simulink library "mcp2515lib"  (R2018b)
settings: Solver=VariableStepAuto  StartTime=0.0  StopTime=10.0  RelTol=1e-3  EnableMultiTasking=on
libraries: $bdroot x33, simulink x26, arduinolib x9, raspberrypilib x9
(part 1 of 2)
settings Model: Creator=ayasuda  LastModifiedBy=Tatsuya Ishikawa
settings DataIOCC: LimitDataPoints=on
settings OptimizationCC: LifeSpan=inf
settings DebuggingCC: UnderspecifiedInitializationDetection=Classic  MergeDetectMultiDrivingBlocksExec=none  AllowSymbolicDim=off  SFUnexpectedBacktrackingDiag=warning  SFNoUnconditionalDefaultTransitionDiag=warning  SFExecutionAtInitializationDiag=none
settings ModelReferenceCC: PropagateSignalLabelsOutOfModel=off
settings SFSimCC: SimUseLocalCustomCode=off
settings RTWCC: RTWUseLocalCustomCode=off
settings CodeAppCC: StateflowObjectComments=on
settings GRTTargetCC: TargetLangStandard=C89/C90 (ANSI)
settings ConfigComp: CovMetricSettings=dw  CovHtmlReporting=on  CovSaveCumulativeToWorkspaceVar=on  CovSaveSingleToWorkspaceVar=on  CovExternalEMLEnable=off

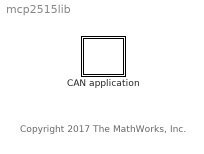
== system mcp2515lib ==
  note: Copyright 2017 The MathWorks, Inc.
  CAN application : Subsystem

== system mcp2515lib/CAN application ==
  note: Copyright 2017 The MathWorks, Inc.
  CANbegin : Subsystem  TreatAsAtomicUnit=on  mask{TargetHardware=Arduino, Oscillator=16, CANSpeed=1000, CSpin=10}
      mask prompts: TargetHardware "Target Hardware"; Oscillator "Oscillator frequency(MHz)"; CANSpeed "CAN speed(kHz)"; CSpin "Chip Select Pin"
      mask init:
      | % Get this mask's handle
      | maskObj = Simulink.Mask.get(gcb);
      | 
      | % Get the selected value from mask parameter's option
      | str_TargetHard = char(maskObj.Parameters(1).TypeOptions(TargetHardware));
      | str_Osc = char(maskObj.Parameters(2).TypeOptions(Oscillator));
      | str_CANSpeed = char(maskObj.Parameters(3).TypeOptions(CANSpeed));
      | 
      | % Set Icon
      | str1 = sprintf('%s(Model)',str_TargetHard);
      | str2 = sprintf('Oscillator: %s(MHz)',str_Osc);
      | str3 = sprintf('CAN Bus Speed: %s(kHz)',str_CANSpeed);
      | str4 = sprintf('Chip Select pin: %d',CSpin);
      | 
      | % Set the values of Variant Subsystem
      | switch str_TargetHard
      |     case 'Arduino'
      |         str = [str1,'\n',str2,'\n',str3,'\n',str4];
      |         evalin('base',sprintf('CSpin = %d;',CSpin));        
      |         evalin('base','Hardware = 1;');
      |     case 'Raspberry Pi'
      |         str = [str1,'\n',str2,'\n',str3];
      |         evalin('base',sprintf('clear CSpin',CSpin));           
      |         evalin('base','Hardware = 2;');     
      | end  
      | 
      | % Get the CAN Configuration register's value from mask parameter's option
      | if str_Osc == '8' %[MHz]
      |     switch str_CANSpeed
      |         case '1000'
      |             BPR = 0; PHSEG1 = 0; PRSEG = 0; PHSEG2 = 0;
      |         case '500'
      |             BPR = 0; PHSEG1 = 2; PRSEG = 0; PHSEG2 = 2;
      |         case '250'
      |             BPR = 0; PHSEG1 = 6; PRSEG = 0; PHSEG2 = 6;
      |         case '125'
      |             BPR = 1; PHSEG1 = 6; PRSEG = 1; PHSEG2 = 5;
      |         case '100'
      |             BPR = 1; PHSEG1 = 7; PRSEG = 2; PHSEG2 = 7;
      |         case '83.3'
      |             BPR = 1; PHSEG1 = 7; PRSEG = 6; PHSEG2 = 7;
      |         case '62.5'
      |             BPR = 3; PHSEG1 = 6; PRSEG = 0; PHSEG2 = 6;
      |         case '50'
      |             BPR = 3; PHSEG1 = 7; PRSEG = 2; PHSEG2 = 7;
      |         case '33.3'
      |             BPR = 4; PHSEG1 = 7; PRSEG = 6; PHSEG2 = 7;
      |     end            
      | elseif str_Osc == '16' %[MHz]
      |     switch str_CANSpeed  
      |         case '1000'
      |             BPR = 0; PHSEG1 = 2; PRSEG = 0; PHSEG2 = 2;
      |         case '500'
      |             BPR = 0; PHSEG1 = 6; PRSEG = 0; PHSEG2 = 6;
      |         case '250'
      |             BPR = 1; PHSEG1 = 6; PRSEG = 1; PHSEG2 = 5;        
      |         case '125'
      |             BPR = 3; PHSEG1 = 6; PRSEG = 0; PHSEG2 = 6;
      |         case '100'
      |             BPR = 3; PHSEG1 = 7; PRSEG = 2; PHSEG2 = 7;
      |         case '83.3'
      |             BPR = 3; PHSEG1 = 7; PRSEG = 6; PHSEG2 = 7;
      |         case '62.5'
      |             BPR = 7; PHSEG1 = 6; PRSEG = 0; PHSEG2 = 6;
      |         case '50'
      |             BPR = 7; PHSEG1 = 7; PRSEG = 2; PHSEG2 = 7;
      |         case '33.3'
      |             BPR = 9; PHSEG1 = 7; PRSEG = 6; PHSEG2 = 7;        
      |     end   
      | end
      | % Set the CAN Configuration register's value
      | address2A = BPR;          % bit7-6 :SJW, bit5-0: BPR
      | address29 = 192 ...       % bit7: BTLMODE = 1, bit6:SAM = 1
      |             + 8*PHSEG1 ...% bit5-3: PHSEG1
      |             +PRSEG;       % bit2-0: PRSEG
      | address28 = 128 ...       % bit7: SOF = 1, bit6:WAKFIL = 0
      |             + PHSEG2;     % bit5-3: 0, bit2-0: PHSEG2
      settings: OpenFcn=open_system(gcbh,'force')  RTWSystemCode=Nonreusable function
      settings: CopyFcn=|
      | set_param(gcbh,'LinkStatus','none');
      | set_param(gcbh,'OpenFcn','');
      | set_param(gcbh,'CopyFcn','')
      mask TypeOptions TargetHardware: Arduino | Raspberry Pi
      mask Callback TargetHardware:
      | if(strcmp(get_param(gcb,'TargetHardware'),'Arduino'))
      |     set_param(gcb,'MaskVisibilities',{'on','on','on','on'})
      | else
      |     set_param(gcb,'MaskVisibilities',{'on','on','on','off'})
      | end
      mask TypeOptions Oscillator: 8 | 16
      mask TypeOptions CANSpeed: 1000 | 500 | 250 | 125 | 100 | 83.3 | 62.5 | 50 | 33.3
      mask DialogControl DescGroupVar Prompt: Description
      mask DialogControl DescTextVar Prompt: This block must be executed only once when beginning CAN communication because MCP2515’s register needs to be configured. And the frequency of oscillator for MCP2515 is also needed because it effects to the setting parameters of MCP2515's register.
      mask Display: disp(str)
  CANbegin CE1 : Subsystem  TreatAsAtomicUnit=on  mask{TargetHardware=Arduino, Oscillator=8, CANSpeed=1000, CSpin=10}
      mask prompts: TargetHardware "Target Hardware"; Oscillator "Oscillator frequency(MHz)"; CANSpeed "CAN speed(kHz)"; CSpin "Chip Select Pin"
      mask init: same as mcp2515lib/CAN application/CANbegin
      settings: OpenFcn=open_system(gcbh,'force')  RTWSystemCode=Nonreusable function
      settings: CopyFcn=|
      | set_param(gcbh,'LinkStatus','none');
      | set_param(gcbh,'OpenFcn','');
      | set_param(gcbh,'CopyFcn','')
      mask TypeOptions TargetHardware: Arduino | Raspberry Pi
      mask Callback TargetHardware:
      | if(strcmp(get_param(gcb,'TargetHardware'),'Arduino'))
      |     set_param(gcb,'MaskVisibilities',{'on','on','on','on'})
      | else
      |     set_param(gcb,'MaskVisibilities',{'on','on','on','off'})
      | end
      mask TypeOptions Oscillator: 8 | 16
      mask TypeOptions CANSpeed: 1000 | 500 | 250 | 125 | 100 | 83.3 | 62.5 | 50 | 33.3
      mask DialogControl DescGroupVar Prompt: Description
      mask DialogControl DescTextVar Prompt: This block must be executed only once when beginning CAN communication because MCP2515’s register needs to be configured. And the frequency of oscillator for MCP2515 is also needed because it effects to the setting parameters of MCP2515's register.
      mask Display: disp(str)
  CANreceive : Subsystem  TreatAsAtomicUnit=on
      settings: OpenFcn=open_system(gcbh,'force')
      settings: CopyFcn=|
      | set_param(gcbh,'LinkStatus','none');
      | set_param(gcbh,'OpenFcn','');
      | set_param(gcbh,'CopyFcn','')
      mask DialogControl DescGroupVar Prompt: Description
      mask DialogControl DescTextVar Prompt: CANreceive outputs CAN data by converting MCP2515 RX buffer register’s values. In/Out ports are no use because they are used for controlling the execution order. CAN_Received outputs 1(CAN received) or -1( No message).
  CANreceive CE1 : Subsystem  TreatAsAtomicUnit=on
      settings: OpenFcn=open_system(gcbh,'force')
      settings: CopyFcn=|
      | set_param(gcbh,'LinkStatus','none');
      | set_param(gcbh,'OpenFcn','');
      | set_param(gcbh,'CopyFcn','')
      mask DialogControl DescGroupVar Prompt: Description
      mask DialogControl DescTextVar Prompt: CANreceive outputs CAN data by converting MCP2515 RX buffer register’s values. In/Out ports are no use because they are used for controlling the execution order. CAN_Received outputs 1(CAN received) or -1( No message).
  CANtransmit : Subsystem  TreatAsAtomicUnit=on
      settings: OpenFcn=open_system(gcbh,'force')
      settings: CopyFcn=|
      | set_param(gcbh,'LinkStatus','none');
      | set_param(gcbh,'OpenFcn','');
      | set_param(gcbh,'CopyFcn','')
      mask DialogControl DescGroupVar Prompt: Description
      mask DialogControl DescTextVar Prompt: CANtransmit inputs CAN data by converting MCP2515 TX buffer register’s values. In/Out ports are no use because they are used for controlling the execution order. CAN_Transmitted outputs 1(Success) or 2(Fail).
  CANtransmit CE1 : Subsystem  TreatAsAtomicUnit=on
      settings: OpenFcn=open_system(gcbh,'force')
      settings: CopyFcn=|
      | set_param(gcbh,'LinkStatus','none');
      | set_param(gcbh,'OpenFcn','');
      | set_param(gcbh,'CopyFcn','')
      mask DialogControl DescGroupVar Prompt: Description
      mask DialogControl DescTextVar Prompt: CANtransmit inputs CAN data by converting MCP2515 TX buffer register’s values. In/Out ports are no use because they are used for controlling the execution order. CAN_Transmitted outputs 1(Success) or 2(Fail).
  mcp2515 driver : Subsystem
  mcp2515 driver CE1 : Subsystem

== system mcp2515lib/CAN application/CANbegin ==
  Constant : Constant  Value=0  OutDataTypeStr=boolean  SampleTime=-1
  Temporary buffer : DataStoreMemory  DataStoreName=temp_1byte  ReadBeforeWriteMsg=warning  WriteAfterWriteMsg=warning  WriteAfterReadMsg=warning  ShowAdditionalParam=off  OutDataTypeStr=uint8
  Unit Delay : UnitDelay  InitialCondition=1  SampleTime=-1
  setup : Subsystem  TreatAsAtomicUnit=on
      settings: RTWSystemCode=Nonreusable function  RTWFileNameOpts=Use subsystem name
  wires:
  Constant/1 -> Unit Delay/1
  Unit Delay/1 -> setup/Enable

== system mcp2515lib/CAN application/CANbegin CE1 ==
  Constant : Constant  Value=0  OutDataTypeStr=boolean  SampleTime=-1
  Temporary buffer : DataStoreMemory  DataStoreName=temp_1byte  ReadBeforeWriteMsg=warning  WriteAfterWriteMsg=warning  WriteAfterReadMsg=warning  ShowAdditionalParam=off  OutDataTypeStr=uint8
  Unit Delay : UnitDelay  InitialCondition=1  SampleTime=-1
  setup : Subsystem  TreatAsAtomicUnit=on
      settings: RTWSystemCode=Nonreusable function  RTWFileNameOpts=Use subsystem name
  wires:
  Constant/1 -> Unit Delay/1
  Unit Delay/1 -> setup/Enable

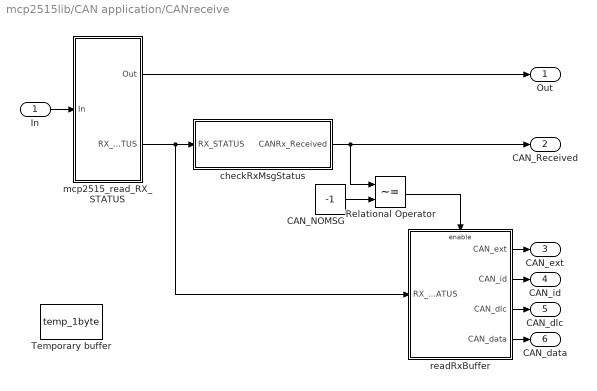
== system mcp2515lib/CAN application/CANreceive ==
  In : Inport
  CAN_NOMSG : Constant  Value=-1  OutDataTypeStr=int8
  Relational Operator : RelationalOperator  Operator=~=  OutDataTypeStr=boolean  RndMeth=Nearest
  Temporary buffer : DataStoreMemory  DataStoreName=temp_1byte  ReadBeforeWriteMsg=warning  WriteAfterWriteMsg=warning  WriteAfterReadMsg=warning  ShowAdditionalParam=off  OutDataTypeStr=uint8
  checkRxMsgStatus : Subsystem  TreatAsAtomicUnit=on
  mcp2515_read_RX_STATUS : Subsystem  TreatAsAtomicUnit=on
  readRxBuffer : Subsystem  TreatAsAtomicUnit=on
  Out : Outport
  CAN_Received : Outport  Port=2
  CAN_ext : Outport  Port=3
  CAN_id : Outport  Port=4
  CAN_dlc : Outport  Port=5
  CAN_data : Outport  Port=6
  wires:
  Relational Operator/1 -> readRxBuffer/Enable
  CAN_NOMSG/1 -> Relational Operator/2
  readRxBuffer/4(CAN_data) -> CAN_data/1
  readRxBuffer/3(CAN_dlc) -> CAN_dlc/1
  readRxBuffer/2(CAN_id) -> CAN_id/1
  readRxBuffer/1(CAN_ext) -> CAN_ext/1
  mcp2515_read_RX_STATUS/2(RX_STATUS) -> checkRxMsgStatus/1(RX_STATUS), readRxBuffer/1(RX_STATUS)
  checkRxMsgStatus/1(CANRx_Received) -> Relational Operator/1, CAN_Received/1
  mcp2515_read_RX_STATUS/1(Out) -> Out/1
  In/1 -> mcp2515_read_RX_STATUS/1(In)

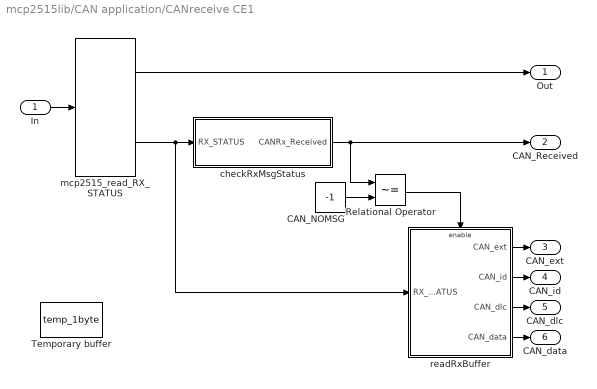
== system mcp2515lib/CAN application/CANreceive CE1 ==
  In : Inport
  CAN_NOMSG : Constant  Value=-1  OutDataTypeStr=int8
  Relational Operator : RelationalOperator  Operator=~=  OutDataTypeStr=boolean  RndMeth=Nearest
  Temporary buffer : DataStoreMemory  DataStoreName=temp_1byte  ReadBeforeWriteMsg=warning  WriteAfterWriteMsg=warning  WriteAfterReadMsg=warning  ShowAdditionalParam=off  OutDataTypeStr=uint8
  checkRxMsgStatus : Subsystem  TreatAsAtomicUnit=on
  mcp2515_read_RX_STATUS : $bdroot/CAN application/mcp2515 driver CE1/mcp2515_read_RX_STATUS  SystemSampleTime=-1
  readRxBuffer : Subsystem  TreatAsAtomicUnit=on
  Out : Outport
  CAN_Received : Outport  Port=2
  CAN_ext : Outport  Port=3
  CAN_id : Outport  Port=4
  CAN_dlc : Outport  Port=5
  CAN_data : Outport  Port=6
  wires:
  Relational Operator/1 -> readRxBuffer/Enable
  CAN_NOMSG/1 -> Relational Operator/2
  readRxBuffer/4(CAN_data) -> CAN_data/1
  readRxBuffer/3(CAN_dlc) -> CAN_dlc/1
  readRxBuffer/2(CAN_id) -> CAN_id/1
  readRxBuffer/1(CAN_ext) -> CAN_ext/1
  mcp2515_read_RX_STATUS/2 -> checkRxMsgStatus/1(RX_STATUS), readRxBuffer/1(RX_STATUS)
  checkRxMsgStatus/1(CANRx_Received) -> Relational Operator/1, CAN_Received/1
  mcp2515_read_RX_STATUS/1 -> Out/1
  In/1 -> mcp2515_read_RX_STATUS/1

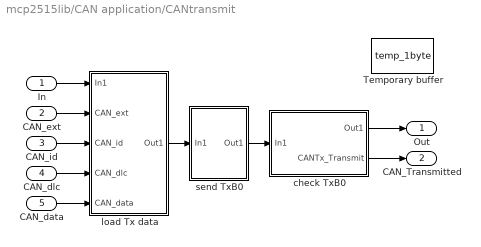
== system mcp2515lib/CAN application/CANtransmit ==
  In : Inport
  CAN_ext : Inport  Port=2
  CAN_id : Inport  Port=3
  CAN_dlc : Inport  Port=4
  CAN_data : Inport  Port=5
  Temporary buffer : DataStoreMemory  DataStoreName=temp_1byte  ReadBeforeWriteMsg=warning  WriteAfterWriteMsg=warning  WriteAfterReadMsg=warning  ShowAdditionalParam=off  OutDataTypeStr=uint8
  check TxB0 : Subsystem  TreatAsAtomicUnit=on
  load Tx data : Subsystem  TreatAsAtomicUnit=on
  send TxB0 : Subsystem  TreatAsAtomicUnit=on
  Out : Outport
  CAN_Transmitted : Outport  Port=2
  wires:
  CAN_data/1 -> load Tx data/5(CAN_data)
  CAN_dlc/1 -> load Tx data/4(CAN_dlc)
  CAN_id/1 -> load Tx data/3(CAN_id)
  CAN_ext/1 -> load Tx data/2(CAN_ext)
  check TxB0/2(CANTx_Transmit) -> CAN_Transmitted/1
  check TxB0/1(Out1) -> Out/1
  send TxB0/1(Out1) -> check TxB0/1(In1)
  load Tx data/1(Out1) -> send TxB0/1(In1)
  In/1 -> load Tx data/1(In1)

== system mcp2515lib/CAN application/CANtransmit CE1 ==
  In : Inport
  CAN_ext : Inport  Port=2
  CAN_id : Inport  Port=3
  CAN_dlc : Inport  Port=4
  CAN_data : Inport  Port=5
  Temporary buffer : DataStoreMemory  DataStoreName=temp_1byte  ReadBeforeWriteMsg=warning  WriteAfterWriteMsg=warning  WriteAfterReadMsg=warning  ShowAdditionalParam=off  OutDataTypeStr=uint8
  check TxB0 : Subsystem  TreatAsAtomicUnit=on
  load Tx data : Subsystem  TreatAsAtomicUnit=on
  send TxB0 : Subsystem  TreatAsAtomicUnit=on
  Out : Outport
  CAN_Transmitted : Outport  Port=2
  wires:
  CAN_data/1 -> load Tx data/5(CAN_data)
  CAN_dlc/1 -> load Tx data/4(CAN_dlc)
  CAN_id/1 -> load Tx data/3(CAN_id)
  CAN_ext/1 -> load Tx data/2(CAN_ext)
  check TxB0/2(CANTx_Transmit) -> CAN_Transmitted/1
  check TxB0/1(Out1) -> Out/1
  send TxB0/1(Out1) -> check TxB0/1(In1)
  load Tx data/1(Out1) -> send TxB0/1(In1)
  In/1 -> load Tx data/1(In1)

== system mcp2515lib/CAN application/mcp2515 driver ==
  SPI driver : Subsystem  Variant=on
      settings: OpenFcn=open_system(gcbh,'force')
  mcp2515_modifyRegister : Subsystem  TreatAsAtomicUnit=on
      settings: OpenFcn=open_system(gcbh,'force')
      settings: CopyFcn=|
      | set_param(gcbh,'LinkStatus','none');
      | set_param(gcbh,'OpenFcn','');
      | set_param(gcbh,'CopyFcn','')
  mcp2515_readRegister : Subsystem  TreatAsAtomicUnit=on
      settings: OpenFcn=open_system(gcbh,'force')
      settings: CopyFcn=|
      | set_param(gcbh,'LinkStatus','none');
      | set_param(gcbh,'OpenFcn','');
      | set_param(gcbh,'CopyFcn','')
  mcp2515_readRxBuffer : Subsystem  TreatAsAtomicUnit=on
      settings: OpenFcn=open_system(gcbh,'force')
      settings: CopyFcn=|
      | set_param(gcbh,'LinkStatus','none');
      | set_param(gcbh,'OpenFcn','');
      | set_param(gcbh,'CopyFcn','')
  mcp2515_read_RX_STATUS : Subsystem  TreatAsAtomicUnit=on
      settings: OpenFcn=open_system(gcbh,'force')
      settings: CopyFcn=|
      | set_param(gcbh,'LinkStatus','none');
      | set_param(gcbh,'OpenFcn','');
      | set_param(gcbh,'CopyFcn','')
  mcp2515_reset : Subsystem  TreatAsAtomicUnit=on
      settings: OpenFcn=open_system(gcbh,'force')
      settings: CopyFcn=|
      | set_param(gcbh,'LinkStatus','none');
      | set_param(gcbh,'OpenFcn','');
      | set_param(gcbh,'CopyFcn','')
  mcp2515_writeRegister : Subsystem  TreatAsAtomicUnit=on
      settings: OpenFcn=open_system(gcbh,'force')
      settings: CopyFcn=|
      | set_param(gcbh,'LinkStatus','none');
      | set_param(gcbh,'OpenFcn','');
      | set_param(gcbh,'CopyFcn','')
  mcp2515_writeTxBuffer : Subsystem  TreatAsAtomicUnit=on
      settings: OpenFcn=open_system(gcbh,'force')
      settings: CopyFcn=|
      | set_param(gcbh,'LinkStatus','none');
      | set_param(gcbh,'OpenFcn','');
      | set_param(gcbh,'CopyFcn','')

== system mcp2515lib/CAN application/mcp2515 driver CE1 ==
  SPI driver : Subsystem  Variant=on
      settings: OpenFcn=open_system(gcbh,'force')
  mcp2515_modifyRegister : Subsystem  TreatAsAtomicUnit=on
  mcp2515_readRegister : Subsystem  TreatAsAtomicUnit=on
  mcp2515_readRxBuffer : Subsystem  TreatAsAtomicUnit=on
  mcp2515_read_RX_STATUS : Subsystem  TreatAsAtomicUnit=on
  mcp2515_reset : Subsystem  TreatAsAtomicUnit=on
  mcp2515_writeRegister : Subsystem  TreatAsAtomicUnit=on
  mcp2515_writeTxBuffer : Subsystem  TreatAsAtomicUnit=on

== system mcp2515lib/CAN application/CANbegin/setup ==
  Enable : EnablePort
  CNF1 : Constant  Value=address2A  OutDataTypeStr=uint8
  CNF2 : Constant  Value=address29  OutDataTypeStr=uint8
  CNF3 : Constant  Value=address28  OutDataTypeStr=uint8
  Ground : Ground
  Terminator : Terminator
  changeCANmode(config) : Subsystem  TreatAsAtomicUnit=on
  changeCANmode(normal) : Subsystem  TreatAsAtomicUnit=on
  mcp2515_reset : Subsystem  TreatAsAtomicUnit=on
  setCANRxBuffer : Subsystem  TreatAsAtomicUnit=on
  setCANspeed : Subsystem  TreatAsAtomicUnit=on
  wires:
  changeCANmode(normal)/1(Out) -> Terminator/1
  Ground/1 -> mcp2515_reset/1(In)
  setCANRxBuffer/1(Out) -> changeCANmode(normal)/1(In)
  setCANspeed/1(Out) -> setCANRxBuffer/1(In)
  changeCANmode(config)/1(Out) -> setCANspeed/1(In)
  mcp2515_reset/1(Out) -> changeCANmode(config)/1(In)
  CNF1/1 -> setCANspeed/2(CNF1)
  CNF2/1 -> setCANspeed/3(CNF2)
  CNF3/1 -> setCANspeed/4(CNF3)

== system mcp2515lib/CAN application/CANbegin CE1/setup ==
  Enable : EnablePort
  CNF1 : Constant  Value=address2A  OutDataTypeStr=uint8
  CNF2 : Constant  Value=address29  OutDataTypeStr=uint8
  CNF3 : Constant  Value=address28  OutDataTypeStr=uint8
  Ground : Ground
  Terminator : Terminator
  changeCANmode(config) : Subsystem  TreatAsAtomicUnit=on
  changeCANmode(normal) : Subsystem  TreatAsAtomicUnit=on
  mcp2515_reset : $bdroot/CAN application/mcp2515 driver CE1/mcp2515_reset  SystemSampleTime=-1
  setCANRxBuffer : Subsystem  TreatAsAtomicUnit=on
  setCANspeed : Subsystem  TreatAsAtomicUnit=on
  wires:
  changeCANmode(normal)/1(Out) -> Terminator/1
  Ground/1 -> mcp2515_reset/1
  setCANRxBuffer/1(Out) -> changeCANmode(normal)/1(In)
  setCANspeed/1(Out) -> setCANRxBuffer/1(In)
  changeCANmode(config)/1(Out) -> setCANspeed/1(In)
  mcp2515_reset/1 -> changeCANmode(config)/1(In)
  CNF1/1 -> setCANspeed/2(CNF1)
  CNF2/1 -> setCANspeed/3(CNF2)
  CNF3/1 -> setCANspeed/4(CNF3)

== system mcp2515lib/CAN application/CANreceive/checkRxMsgStatus ==
  RX_STATUS : Inport
  Bitmask_RxBn : simulink/Logic and Bit Operations/Bitwise Operator  logicop=AND  UseBitMask=on  BitMask=bin2dec('11000000')  BitMaskRealWorld=Stored Integer
  CAN_NOMSG : Constant  Value=-1  OutDataTypeStr=int8
  CAN_OK : Constant  OutDataTypeStr=int8
  Switch : Switch  Criteria=u2 > Threshold
  CANRx_Received : Outport
  wires:
  Bitmask_RxBn/1 -> Switch/2
  Switch/1 -> CANRx_Received/1
  CAN_NOMSG/1 -> Switch/3
  CAN_OK/1 -> Switch/1
  RX_STATUS/1 -> Bitmask_RxBn/1

== system mcp2515lib/CAN application/CANreceive/mcp2515_read_RX_STATUS ==
  In : Inport
  Constant : Constant  Value=0  OutDataTypeStr=uint8
  MCP_RX_STATUS : Constant  Value=hex2dec('B0')  OutDataTypeStr=uint8
  SPI driver : $bdroot/CAN application/mcp2515 driver/SPI driver  SystemSampleTime=-1
  Selector : Selector  IndexMode=Zero-based  InputPortWidth=2  IndexOptions=Index vector (dialog)  Indices=1  OutputSizes=1
  Vector Concatenate : Concatenate
  Out : Outport
  RX_STATUS : Outport  Port=2
  wires:
  Vector Concatenate/1 -> SPI driver/1
  MCP_RX_STATUS/1 -> Vector Concatenate/1
  Selector/1 -> RX_STATUS/1
  SPI driver/1 -> Selector/1
  Constant/1 -> Vector Concatenate/2
  In/1 -> Out/1

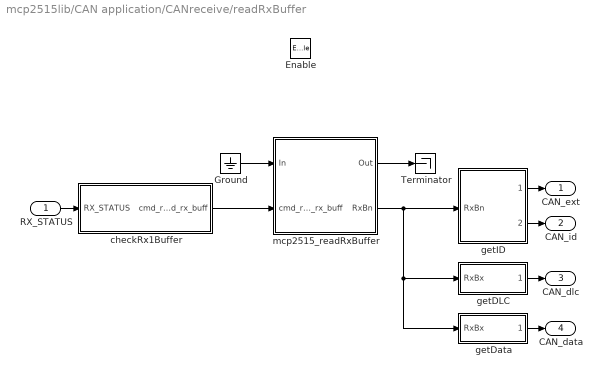
== system mcp2515lib/CAN application/CANreceive/readRxBuffer ==
  RX_STATUS : Inport
  Enable : EnablePort
  Ground : Ground
  Terminator : Terminator
  checkRx1Buffer : Subsystem  TreatAsAtomicUnit=on
  getDLC : Subsystem  TreatAsAtomicUnit=on
  getData : Subsystem  TreatAsAtomicUnit=on
  getID : Subsystem  TreatAsAtomicUnit=on
      settings: RTWSystemCode=Inline
  mcp2515_readRxBuffer : Subsystem  TreatAsAtomicUnit=on
  CAN_ext : Outport
  CAN_id : Outport  Port=2
  CAN_dlc : Outport  Port=3
  CAN_data : Outport  Port=4
  wires:
  checkRx1Buffer/1(cmd_read_rx_buff) -> mcp2515_readRxBuffer/2(cmd_read_rx_buff)
  RX_STATUS/1 -> checkRx1Buffer/1(RX_STATUS)
  Ground/1 -> mcp2515_readRxBuffer/1(In)
  mcp2515_readRxBuffer/1(Out) -> Terminator/1
  getDLC/1(CAN_dlc) -> CAN_dlc/1
  getID/1(CAN_ext) -> CAN_ext/1
  getID/2(CAN_id) -> CAN_id/1
  mcp2515_readRxBuffer/2(RxBn) -> getDLC/1(RxBx), getData/1(RxBx), getID/1(RxBn)
  getData/1(CAN_data) -> CAN_data/1

== system mcp2515lib/CAN application/CANreceive CE1/checkRxMsgStatus ==
  RX_STATUS : Inport
  Bitmask_RxBn : simulink/Logic and Bit Operations/Bitwise Operator  logicop=AND  UseBitMask=on  BitMask=bin2dec('11000000')  BitMaskRealWorld=Stored Integer
  CAN_NOMSG : Constant  Value=-1  OutDataTypeStr=int8
  CAN_OK : Constant  OutDataTypeStr=int8
  Switch : Switch  Criteria=u2 > Threshold
  CANRx_Received : Outport
  wires:
  Bitmask_RxBn/1 -> Switch/2
  Switch/1 -> CANRx_Received/1
  CAN_NOMSG/1 -> Switch/3
  CAN_OK/1 -> Switch/1
  RX_STATUS/1 -> Bitmask_RxBn/1

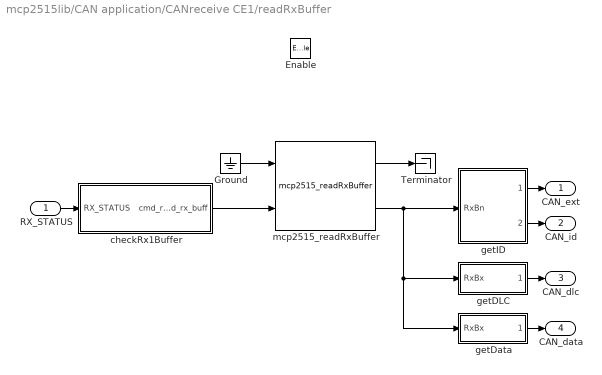
== system mcp2515lib/CAN application/CANreceive CE1/readRxBuffer ==
  RX_STATUS : Inport
  Enable : EnablePort
  Ground : Ground
  Terminator : Terminator
  checkRx1Buffer : Subsystem  TreatAsAtomicUnit=on
  getDLC : Subsystem  TreatAsAtomicUnit=on
  getData : Subsystem  TreatAsAtomicUnit=on
  getID : Subsystem  TreatAsAtomicUnit=on
      settings: RTWSystemCode=Inline
  mcp2515_readRxBuffer : $bdroot/CAN application/mcp2515 driver CE1/mcp2515_readRxBuffer  SystemSampleTime=-1
  CAN_ext : Outport
  CAN_id : Outport  Port=2
  CAN_dlc : Outport  Port=3
  CAN_data : Outport  Port=4
  wires:
  checkRx1Buffer/1(cmd_read_rx_buff) -> mcp2515_readRxBuffer/2
  RX_STATUS/1 -> checkRx1Buffer/1(RX_STATUS)
  Ground/1 -> mcp2515_readRxBuffer/1
  mcp2515_readRxBuffer/1 -> Terminator/1
  getDLC/1(CAN_dlc) -> CAN_dlc/1
  getID/1(CAN_ext) -> CAN_ext/1
  getID/2(CAN_id) -> CAN_id/1
  mcp2515_readRxBuffer/2 -> getDLC/1(RxBx), getData/1(RxBx), getID/1(RxBn)
  getData/1(CAN_data) -> CAN_data/1

== system mcp2515lib/CAN application/CANtransmit/check TxB0 ==
  In1 : Inport
  Bitmask_TxReq : simulink/Logic and Bit Operations/Bitwise Operator  logicop=AND  UseBitMask=on  BitMask=bin2dec('00001000')  BitMaskRealWorld=Stored Integer
  CAN_FAIL : Constant  Value=2  OutDataTypeStr=int8
  CAN_OK : Constant  OutDataTypeStr=int8
  MCP_TxB0CTRL1 : Constant  Value=hex2dec('30')  OutDataTypeStr=uint8
  Switch : Switch  Criteria=u2 > Threshold
  mcp2515_readRegister : Subsystem  TreatAsAtomicUnit=on
  Out1 : Outport
  CANTx_Transmit : Outport  Port=2
  wires:
  In1/1 -> mcp2515_readRegister/1(In)
  CAN_OK/1 -> Switch/1
  Switch/1 -> CANTx_Transmit/1
  Bitmask_TxReq/1 -> Switch/2
  MCP_TxB0CTRL1/1 -> mcp2515_readRegister/2(address)
  mcp2515_readRegister/2(SPI_data) -> Bitmask_TxReq/1
  mcp2515_readRegister/1(Out) -> Out1/1
  CAN_FAIL/1 -> Switch/3

== system mcp2515lib/CAN application/CANtransmit/load Tx data ==
  In1 : Inport
  CAN_ext : Inport  Port=2
  CAN_id : Inport  Port=3
  CAN_dlc : Inport  Port=4
  CAN_data : Inport  Port=5
  MCP_load_TxB0 : Constant  Value=hex2dec('40')  OutDataTypeStr=uint8
  Vector Concatenate : Concatenate  NumInputs=3
  mcp2515_writeTxBuffer : Subsystem  TreatAsAtomicUnit=on
  setID : Subsystem  TreatAsAtomicUnit=on
      settings: RTWSystemCode=Inline
  Out1 : Outport
  wires:
  Vector Concatenate/1 -> mcp2515_writeTxBuffer/3(data_tx_buff)
  MCP_load_TxB0/1 -> mcp2515_writeTxBuffer/2(cmd_load_tx_buff)
  mcp2515_writeTxBuffer/1(Out) -> Out1/1
  In1/1 -> mcp2515_writeTxBuffer/1(In)
  setID/1(TxBn_ID) -> Vector Concatenate/1
  CAN_dlc/1 -> Vector Concatenate/2
  CAN_data/1 -> Vector Concatenate/3
  CAN_id/1 -> setID/2(id)
  CAN_ext/1 -> setID/1(ext)

== system mcp2515lib/CAN application/CANtransmit/send TxB0 ==
  In1 : Inport
  MCP_TxB0CTRL : Constant  Value=hex2dec('30')  OutDataTypeStr=uint8
  TxREQ : Constant  Value=8  OutDataTypeStr=uint8
  mcp2515_writeRegister : Subsystem  TreatAsAtomicUnit=on
  Out1 : Outport
  wires:
  TxREQ/1 -> mcp2515_writeRegister/3(value)
  In1/1 -> mcp2515_writeRegister/1(In)
  mcp2515_writeRegister/1(Out) -> Out1/1
  MCP_TxB0CTRL/1 -> mcp2515_writeRegister/2(address)

== system mcp2515lib/CAN application/CANtransmit CE1/check TxB0 ==
  In1 : Inport
  Bitmask_TxReq : simulink/Logic and Bit Operations/Bitwise Operator  logicop=AND  UseBitMask=on  BitMask=bin2dec('00001000')  BitMaskRealWorld=Stored Integer
  CAN_FAIL : Constant  Value=2  OutDataTypeStr=int8
  CAN_OK : Constant  OutDataTypeStr=int8
  MCP_TxB0CTRL1 : Constant  Value=hex2dec('30')  OutDataTypeStr=uint8
  Switch : Switch  Criteria=u2 > Threshold
  mcp2515_readRegister : $bdroot/CAN application/mcp2515 driver CE1/mcp2515_readRegister  SystemSampleTime=-1
  Out1 : Outport
  CANTx_Transmit : Outport  Port=2
  wires:
  In1/1 -> mcp2515_readRegister/1
  CAN_OK/1 -> Switch/1
  Switch/1 -> CANTx_Transmit/1
  Bitmask_TxReq/1 -> Switch/2
  MCP_TxB0CTRL1/1 -> mcp2515_readRegister/2
  mcp2515_readRegister/2 -> Bitmask_TxReq/1
  mcp2515_readRegister/1 -> Out1/1
  CAN_FAIL/1 -> Switch/3

== system mcp2515lib/CAN application/CANtransmit CE1/load Tx data ==
  In1 : Inport
  CAN_ext : Inport  Port=2
  CAN_id : Inport  Port=3
  CAN_dlc : Inport  Port=4
  CAN_data : Inport  Port=5
  MCP_load_TxB0 : Constant  Value=hex2dec('40')  OutDataTypeStr=uint8
  Vector Concatenate : Concatenate  NumInputs=3
  mcp2515_writeTxBuffer : $bdroot/CAN application/mcp2515 driver CE1/mcp2515_writeTxBuffer  SystemSampleTime=-1
  setID : Subsystem  TreatAsAtomicUnit=on
      settings: RTWSystemCode=Inline
  Out1 : Outport
  wires:
  Vector Concatenate/1 -> mcp2515_writeTxBuffer/3
  MCP_load_TxB0/1 -> mcp2515_writeTxBuffer/2
  mcp2515_writeTxBuffer/1 -> Out1/1
  In1/1 -> mcp2515_writeTxBuffer/1
  setID/1(TxBn_ID) -> Vector Concatenate/1
  CAN_dlc/1 -> Vector Concatenate/2
  CAN_data/1 -> Vector Concatenate/3
  CAN_id/1 -> setID/2(id)
  CAN_ext/1 -> setID/1(ext)

== system mcp2515lib/CAN application/CANtransmit CE1/send TxB0 ==
  In1 : Inport
  MCP_TxB0CTRL : Constant  Value=hex2dec('30')  OutDataTypeStr=uint8
  TxREQ : Constant  Value=8  OutDataTypeStr=uint8
  mcp2515_writeRegister1 : $bdroot/CAN application/mcp2515 driver CE1/mcp2515_writeRegister  SystemSampleTime=-1
  Out1 : Outport
  wires:
  TxREQ/1 -> mcp2515_writeRegister1/3
  In1/1 -> mcp2515_writeRegister1/1
  mcp2515_writeRegister1/1 -> Out1/1
  MCP_TxB0CTRL/1 -> mcp2515_writeRegister1/2

== system mcp2515lib/CAN application/mcp2515 driver/SPI driver ==
  SPIdata_In : Inport
  Arduino : Subsystem  TreatAsAtomicUnit=on  VariantControl=Hardware == 1
  Rapberry Pi : Subsystem  TreatAsAtomicUnit=on  VariantControl=Hardware == 2
  SPIdata_Out : Outport

== system mcp2515lib/CAN application/mcp2515 driver/mcp2515_modifyRegister ==
  In : Inport
  address : Inport  Port=2
  mask : Inport  Port=3
  data : Inport  Port=4
  MCP_BITMOD : Constant  Value=5  OutDataTypeStr=uint8
  SPI driver : $bdroot/CAN application/mcp2515 driver/SPI driver  SystemSampleTime=-1
  Selector : Selector  IndexMode=Zero-based  InputPortWidth=4  IndexOptions=Index vector (dialog)  Indices=0  OutputSizes=1
  Temporary buffer : DataStoreWrite  DataStoreName=temp_1byte
  Vector Concatenate : Concatenate  NumInputs=4
  Out : Outport
  wires:
  SPI driver/1 -> Selector/1
  data/1 -> Vector Concatenate/4
  address/1 -> Vector Concatenate/2
  mask/1 -> Vector Concatenate/3
  MCP_BITMOD/1 -> Vector Concatenate/1
  In/1 -> Out/1
  Selector/1 -> Temporary buffer/1
  Vector Concatenate/1 -> SPI driver/1

== system mcp2515lib/CAN application/mcp2515 driver/mcp2515_readRegister ==
  In : Inport
  address : Inport  Port=2  OutDataTypeStr=uint8
  Constant : Constant  Value=0  OutDataTypeStr=uint8
  MCP_READ : Constant  Value=3  OutDataTypeStr=uint8
  SPI driver : $bdroot/CAN application/mcp2515 driver/SPI driver  SystemSampleTime=-1
  Selector : Selector  IndexMode=Zero-based  InputPortWidth=3  IndexOptions=Index vector (dialog)  Indices=2  OutputSizes=1
  Vector Concatenate : Concatenate  NumInputs=3
  Out : Outport
  SPI_data : Outport  Port=2
  wires:
  SPI driver/1 -> Selector/1
  address/1 -> Vector Concatenate/2
  Constant/1 -> Vector Concatenate/3
  In/1 -> Out/1
  MCP_READ/1 -> Vector Concatenate/1
  Selector/1 -> SPI_data/1
  Vector Concatenate/1 -> SPI driver/1

== system mcp2515lib/CAN application/mcp2515 driver/mcp2515_readRxBuffer ==
  In : Inport
  cmd_read_rx_buff : Inport  Port=2
  Constant : Constant  Value=zeros(1,13)  OutDataTypeStr=uint8
  SPI driver : $bdroot/CAN application/mcp2515 driver/SPI driver  SystemSampleTime=-1
  Selector1 : Selector  IndexMode=Zero-based  InputPortWidth=14  IndexOptions=Index vector (dialog)  Indices=[1:13]  OutputSizes=1
  Vector Concatenate : Concatenate
  Out : Outport
  RxBn : Outport  Port=2
  wires:
  cmd_read_rx_buff/1 -> Vector Concatenate/1
  Constant/1 -> Vector Concatenate/2
  Vector Concatenate/1 -> SPI driver/1
  SPI driver/1 -> Selector1/1
  Selector1/1 -> RxBn/1
  In/1 -> Out/1

== system mcp2515lib/CAN application/mcp2515 driver/mcp2515_read_RX_STATUS ==
  In : Inport
  Constant : Constant  Value=0  OutDataTypeStr=uint8
  MCP_RX_STATUS : Constant  Value=hex2dec('B0')  OutDataTypeStr=uint8
  SPI driver : $bdroot/CAN application/mcp2515 driver/SPI driver  SystemSampleTime=-1
  Selector : Selector  IndexMode=Zero-based  InputPortWidth=2  IndexOptions=Index vector (dialog)  Indices=1  OutputSizes=1
  Vector Concatenate : Concatenate
  Out : Outport
  RX_STATUS : Outport  Port=2
  wires:
  In/1 -> Out/1
  Constant/1 -> Vector Concatenate/2
  SPI driver/1 -> Selector/1
  Selector/1 -> RX_STATUS/1
  MCP_RX_STATUS/1 -> Vector Concatenate/1
  Vector Concatenate/1 -> SPI driver/1

== system mcp2515lib/CAN application/mcp2515 driver/mcp2515_reset ==
  In : Inport
  MCP_RESET : Constant  Value=hex2dec('C0')  OutDataTypeStr=uint8
  SPI driver : $bdroot/CAN application/mcp2515 driver/SPI driver  SystemSampleTime=-1
  Temporary buffer : DataStoreWrite  DataStoreName=temp_1byte
  Out : Outport
  wires:
  MCP_RESET/1 -> SPI driver/1
  In/1 -> Out/1
  SPI driver/1 -> Temporary buffer/1

== system mcp2515lib/CAN application/mcp2515 driver/mcp2515_writeRegister ==
  In : Inport
  address : Inport  Port=2  OutDataTypeStr=uint8
  value : Inport  Port=3  OutDataTypeStr=uint8
  MCP_WRITE : Constant  Value=2  OutDataTypeStr=uint8
  SPI driver : $bdroot/CAN application/mcp2515 driver/SPI driver  SystemSampleTime=-1
  Selector : Selector  IndexMode=Zero-based  InputPortWidth=3  IndexOptions=Index vector (dialog)  Indices=0  OutputSizes=1
  Temporary buffer : DataStoreWrite  DataStoreName=temp_1byte
  Vector Concatenate : Concatenate  NumInputs=3
  Out : Outport
  wires:
  SPI driver/1 -> Selector/1
  Selector/1 -> Temporary buffer/1
  In/1 -> Out/1
  Vector Concatenate/1 -> SPI driver/1
  value/1 -> Vector Concatenate/3
  address/1 -> Vector Concatenate/2
  MCP_WRITE/1 -> Vector Concatenate/1

== system mcp2515lib/CAN application/mcp2515 driver/mcp2515_writeTxBuffer ==
  In : Inport
  cmd_load_tx_buff : Inport  Port=2
  data_tx_buff : Inport  Port=3
  SPI driver : $bdroot/CAN application/mcp2515 driver/SPI driver  SystemSampleTime=-1
  Selector1 : Selector  IndexMode=Zero-based  InputPortWidth=14  IndexOptions=Index vector (dialog)  Indices=0  OutputSizes=1
  Temporary buffer : DataStoreWrite  DataStoreName=temp_1byte
  Vector Concatenate : Concatenate
  Out : Outport
  wires:
  In/1 -> Out/1
  SPI driver/1 -> Selector1/1
  data_tx_buff/1 -> Vector Concatenate/2
  cmd_load_tx_buff/1 -> Vector Concatenate/1
  Selector1/1 -> Temporary buffer/1
  Vector Concatenate/1 -> SPI driver/1

== system mcp2515lib/CAN application/mcp2515 driver CE1/SPI driver ==
  SPIdata_In : Inport
  Arduino : Subsystem  TreatAsAtomicUnit=on  VariantControl=Hardware == 1
  Rapberry Pi : Subsystem  TreatAsAtomicUnit=on  VariantControl=Hardware == 2
  SPIdata_Out : Outport

== system mcp2515lib/CAN application/mcp2515 driver CE1/mcp2515_modifyRegister ==
  In : Inport
  address : Inport  Port=2
  mask : Inport  Port=3
  data : Inport  Port=4
  MCP_BITMOD : Constant  Value=5  OutDataTypeStr=uint8
  SPI driver : Subsystem  Variant=on
      settings: OpenFcn=open_system(gcbh,'force')
  Selector : Selector  IndexMode=Zero-based  InputPortWidth=4  IndexOptions=Index vector (dialog)  Indices=0  OutputSizes=1
  Temporary buffer : DataStoreWrite  DataStoreName=temp_1byte
  Vector Concatenate : Concatenate  NumInputs=4
  Out : Outport
  wires:
  SPI driver/1(SPIdata_Out) -> Selector/1
  data/1 -> Vector Concatenate/4
  address/1 -> Vector Concatenate/2
  mask/1 -> Vector Concatenate/3
  MCP_BITMOD/1 -> Vector Concatenate/1
  In/1 -> Out/1
  Selector/1 -> Temporary buffer/1
  Vector Concatenate/1 -> SPI driver/1(SPIdata_In)

== system mcp2515lib/CAN application/mcp2515 driver CE1/mcp2515_readRegister ==
  In : Inport
  address : Inport  Port=2  OutDataTypeStr=uint8
  Constant : Constant  Value=0  OutDataTypeStr=uint8
  MCP_READ : Constant  Value=3  OutDataTypeStr=uint8
  SPI driver : Subsystem  Variant=on
      settings: OpenFcn=open_system(gcbh,'force')
  Selector : Selector  IndexMode=Zero-based  InputPortWidth=3  IndexOptions=Index vector (dialog)  Indices=2  OutputSizes=1
  Vector Concatenate : Concatenate  NumInputs=3
  Out : Outport
  SPI_data : Outport  Port=2
  wires:
  SPI driver/1(SPIdata_Out) -> Selector/1
  address/1 -> Vector Concatenate/2
  Constant/1 -> Vector Concatenate/3
  In/1 -> Out/1
  MCP_READ/1 -> Vector Concatenate/1
  Selector/1 -> SPI_data/1
  Vector Concatenate/1 -> SPI driver/1(SPIdata_In)

== system mcp2515lib/CAN application/mcp2515 driver CE1/mcp2515_readRxBuffer ==
  In : Inport
  cmd_read_rx_buff : Inport  Port=2
  Constant : Constant  Value=zeros(1,13)  OutDataTypeStr=uint8
  SPI driver : Subsystem  Variant=on
      settings: OpenFcn=open_system(gcbh,'force')
  Selector1 : Selector  IndexMode=Zero-based  InputPortWidth=14  IndexOptions=Index vector (dialog)  Indices=[1:13]  OutputSizes=1
  Vector Concatenate : Concatenate
  Out : Outport
  RxBn : Outport  Port=2
  wires:
  cmd_read_rx_buff/1 -> Vector Concatenate/1
  Constant/1 -> Vector Concatenate/2
  Vector Concatenate/1 -> SPI driver/1(SPIdata_In)
  SPI driver/1(SPIdata_Out) -> Selector1/1
  Selector1/1 -> RxBn/1
  In/1 -> Out/1

== system mcp2515lib/CAN application/mcp2515 driver CE1/mcp2515_read_RX_STATUS ==
  In : Inport
  Constant : Constant  Value=0  OutDataTypeStr=uint8
  MCP_RX_STATUS : Constant  Value=hex2dec('B0')  OutDataTypeStr=uint8
  SPI driver : Subsystem  Variant=on
      settings: OpenFcn=open_system(gcbh,'force')
  Selector : Selector  IndexMode=Zero-based  InputPortWidth=2  IndexOptions=Index vector (dialog)  Indices=1  OutputSizes=1
  Vector Concatenate : Concatenate
  Out : Outport
  RX_STATUS : Outport  Port=2
  wires:
  In/1 -> Out/1
  Constant/1 -> Vector Concatenate/2
  SPI driver/1(SPIdata_Out) -> Selector/1
  Selector/1 -> RX_STATUS/1
  MCP_RX_STATUS/1 -> Vector Concatenate/1
  Vector Concatenate/1 -> SPI driver/1(SPIdata_In)

== system mcp2515lib/CAN application/mcp2515 driver CE1/mcp2515_reset ==
  In : Inport
  MCP_RESET : Constant  Value=hex2dec('C0')  OutDataTypeStr=uint8
  SPI driver : Subsystem  Variant=on
      settings: OpenFcn=open_system(gcbh,'force')
  Temporary buffer : DataStoreWrite  DataStoreName=temp_1byte
  Out : Outport
  wires:
  MCP_RESET/1 -> SPI driver/1(SPIdata_In)
  In/1 -> Out/1
  SPI driver/1(SPIdata_Out) -> Temporary buffer/1

== system mcp2515lib/CAN application/mcp2515 driver CE1/mcp2515_writeRegister ==
  In : Inport
  address : Inport  Port=2  OutDataTypeStr=uint8
  value : Inport  Port=3  OutDataTypeStr=uint8
  MCP_WRITE : Constant  Value=2  OutDataTypeStr=uint8
  SPI driver : Subsystem  Variant=on
      settings: OpenFcn=open_system(gcbh,'force')
  Selector : Selector  IndexMode=Zero-based  InputPortWidth=3  IndexOptions=Index vector (dialog)  Indices=0  OutputSizes=1
  Temporary buffer : DataStoreWrite  DataStoreName=temp_1byte
  Vector Concatenate : Concatenate  NumInputs=3
  Out : Outport
  wires:
  SPI driver/1(SPIdata_Out) -> Selector/1
  Selector/1 -> Temporary buffer/1
  In/1 -> Out/1
  Vector Concatenate/1 -> SPI driver/1(SPIdata_In)
  value/1 -> Vector Concatenate/3
  address/1 -> Vector Concatenate/2
  MCP_WRITE/1 -> Vector Concatenate/1

== system mcp2515lib/CAN application/mcp2515 driver CE1/mcp2515_writeTxBuffer ==
  In : Inport
  cmd_load_tx_buff : Inport  Port=2
  data_tx_buff : Inport  Port=3
  SPI driver : Subsystem  Variant=on
      settings: OpenFcn=open_system(gcbh,'force')
  Selector1 : Selector  IndexMode=Zero-based  InputPortWidth=14  IndexOptions=Index vector (dialog)  Indices=0  OutputSizes=1
  Temporary buffer : DataStoreWrite  DataStoreName=temp_1byte
  Vector Concatenate : Concatenate
  Out : Outport
  wires:
  In/1 -> Out/1
  SPI driver/1(SPIdata_Out) -> Selector1/1
  data_tx_buff/1 -> Vector Concatenate/2
  cmd_load_tx_buff/1 -> Vector Concatenate/1
  Selector1/1 -> Temporary buffer/1
  Vector Concatenate/1 -> SPI driver/1(SPIdata_In)

== system mcp2515lib/CAN application/CANbegin/setup/changeCANmode(config) ==
  In : Inport
  MCP_CANCTRL : Constant  Value=hex2dec('0F')  OutDataTypeStr=uint8
  MODE_CONFIG : Constant  Value=hex2dec('80')  OutDataTypeStr=uint8
  MODE_MASK : Constant  Value=hex2dec('E0')  OutDataTypeStr=uint8
  mcp2515_modifyRegister : Subsystem  TreatAsAtomicUnit=on
  Out : Outport
  wires:
  mcp2515_modifyRegister/1(Out) -> Out/1
  In/1 -> mcp2515_modifyRegister/1(In)
  MCP_CANCTRL/1 -> mcp2515_modifyRegister/2(address)
  MODE_MASK/1 -> mcp2515_modifyRegister/3(mask)
  MODE_CONFIG/1 -> mcp2515_modifyRegister/4(data)

== system mcp2515lib/CAN application/CANbegin/setup/changeCANmode(normal) ==
  In : Inport
  MCP_CANCTRL : Constant  Value=hex2dec('0F')  OutDataTypeStr=uint8
  MODE_MASK : Constant  Value=hex2dec('E0')  OutDataTypeStr=uint8
  MODE_NORMAL : Constant  Value=0  OutDataTypeStr=uint8
  mcp2515_modifyRegister : Subsystem  TreatAsAtomicUnit=on
  Out : Outport
  wires:
  mcp2515_modifyRegister/1(Out) -> Out/1
  In/1 -> mcp2515_modifyRegister/1(In)
  MCP_CANCTRL/1 -> mcp2515_modifyRegister/2(address)
  MODE_NORMAL/1 -> mcp2515_modifyRegister/4(data)
  MODE_MASK/1 -> mcp2515_modifyRegister/3(mask)

== system mcp2515lib/CAN application/CANbegin/setup/mcp2515_reset ==
  In : Inport
  MCP_RESET : Constant  Value=hex2dec('C0')  OutDataTypeStr=uint8
  SPI driver : $bdroot/CAN application/mcp2515 driver/SPI driver  SystemSampleTime=-1
  Temporary buffer : DataStoreWrite  DataStoreName=temp_1byte
  Out : Outport
  wires:
  SPI driver/1 -> Temporary buffer/1
  In/1 -> Out/1
  MCP_RESET/1 -> SPI driver/1

== system mcp2515lib/CAN application/CANbegin/setup/setCANRxBuffer ==
  note: no filter, no mask
  note: RXB1
  note: RXB0
  In : Inport
  MCP_RXB0CTRL : Constant  Value=hex2dec('60')  OutDataTypeStr=uint8
  MCP_RXB1CTRL : Constant  Value=hex2dec('70')  OutDataTypeStr=uint8
  MCP_RXB_RX_MASK : Constant  Value=hex2dec('60')  OutDataTypeStr=uint8
  mcp2515_writeRegister : Subsystem  TreatAsAtomicUnit=on
  mcp2515_writeRegister1 : Subsystem  TreatAsAtomicUnit=on
  Out : Outport
  wires:
  mcp2515_writeRegister/1(Out) -> mcp2515_writeRegister1/1(In)
  mcp2515_writeRegister1/1(Out) -> Out/1
  In/1 -> mcp2515_writeRegister/1(In)
  MCP_RXB_RX_MASK/1 -> mcp2515_writeRegister/3(value), mcp2515_writeRegister1/3(value)
  MCP_RXB1CTRL/1 -> mcp2515_writeRegister1/2(address)
  MCP_RXB0CTRL/1 -> mcp2515_writeRegister/2(address)

== system mcp2515lib/CAN application/CANbegin/setup/setCANspeed ==
  In : Inport
  CNF1 : Inport  Port=2
  CNF2 : Inport  Port=3
  CNF3 : Inport  Port=4
  MCP_CNF1 : Constant  Value=hex2dec('2A')  OutDataTypeStr=uint8
  MCP_CNF2 : Constant  Value=hex2dec('29')  OutDataTypeStr=uint8
  MCP_CNF3 : Constant  Value=hex2dec('28')  OutDataTypeStr=uint8
  mcp2515_writeRegister1 : Subsystem  TreatAsAtomicUnit=on
  mcp2515_writeRegister2 : Subsystem  TreatAsAtomicUnit=on
  mcp2515_writeRegister3 : Subsystem  TreatAsAtomicUnit=on
  Out : Outport
  wires:
  mcp2515_writeRegister3/1(Out) -> Out/1
  mcp2515_writeRegister2/1(Out) -> mcp2515_writeRegister3/1(In)
  mcp2515_writeRegister1/1(Out) -> mcp2515_writeRegister2/1(In)
  In/1 -> mcp2515_writeRegister1/1(In)
  CNF2/1 -> mcp2515_writeRegister2/3(value)
  MCP_CNF1/1 -> mcp2515_writeRegister1/2(address)
  CNF1/1 -> mcp2515_writeRegister1/3(value)
  CNF3/1 -> mcp2515_writeRegister3/3(value)
  MCP_CNF3/1 -> mcp2515_writeRegister3/2(address)
  MCP_CNF2/1 -> mcp2515_writeRegister2/2(address)

== system mcp2515lib/CAN application/CANbegin CE1/setup/changeCANmode(config) ==
  In : Inport
  MCP_CANCTRL : Constant  Value=hex2dec('0F')  OutDataTypeStr=uint8
  MODE_CONFIG : Constant  Value=hex2dec('80')  OutDataTypeStr=uint8
  MODE_MASK : Constant  Value=hex2dec('E0')  OutDataTypeStr=uint8
  mcp2515_modifyRegister : $bdroot/CAN application/mcp2515 driver CE1/mcp2515_modifyRegister  SystemSampleTime=-1
  Out : Outport
  wires:
  mcp2515_modifyRegister/1 -> Out/1
  In/1 -> mcp2515_modifyRegister/1
  MCP_CANCTRL/1 -> mcp2515_modifyRegister/2
  MODE_MASK/1 -> mcp2515_modifyRegister/3
  MODE_CONFIG/1 -> mcp2515_modifyRegister/4

== system mcp2515lib/CAN application/CANbegin CE1/setup/changeCANmode(normal) ==
  In : Inport
  MCP_CANCTRL : Constant  Value=hex2dec('0F')  OutDataTypeStr=uint8
  MODE_MASK : Constant  Value=hex2dec('E0')  OutDataTypeStr=uint8
  MODE_NORMAL : Constant  Value=0  OutDataTypeStr=uint8
  mcp2515_modifyRegister : $bdroot/CAN application/mcp2515 driver CE1/mcp2515_modifyRegister  SystemSampleTime=-1
  Out : Outport
  wires:
  mcp2515_modifyRegister/1 -> Out/1
  In/1 -> mcp2515_modifyRegister/1
  MCP_CANCTRL/1 -> mcp2515_modifyRegister/2
  MODE_NORMAL/1 -> mcp2515_modifyRegister/4
  MODE_MASK/1 -> mcp2515_modifyRegister/3

== system mcp2515lib/CAN application/CANbegin CE1/setup/setCANRxBuffer ==
  note: no filter, no mask
  note: RXB1
  note: RXB0
  In : Inport
  MCP_RXB0CTRL : Constant  Value=hex2dec('60')  OutDataTypeStr=uint8
  MCP_RXB1CTRL : Constant  Value=hex2dec('70')  OutDataTypeStr=uint8
  MCP_RXB_RX_MASK : Constant  Value=hex2dec('60')  OutDataTypeStr=uint8
  mcp2515_writeRegister : $bdroot/CAN application/mcp2515 driver CE1/mcp2515_writeRegister  SystemSampleTime=-1
  mcp2515_writeRegister1 : $bdroot/CAN application/mcp2515 driver CE1/mcp2515_writeRegister  SystemSampleTime=-1
  Out : Outport
  wires:
  mcp2515_writeRegister/1 -> mcp2515_writeRegister1/1
  mcp2515_writeRegister1/1 -> Out/1
  In/1 -> mcp2515_writeRegister/1
  MCP_RXB_RX_MASK/1 -> mcp2515_writeRegister1/3, mcp2515_writeRegister/3
  MCP_RXB1CTRL/1 -> mcp2515_writeRegister1/2
  MCP_RXB0CTRL/1 -> mcp2515_writeRegister/2

== system mcp2515lib/CAN application/CANbegin CE1/setup/setCANspeed ==
  In : Inport
  CNF1 : Inport  Port=2
  CNF2 : Inport  Port=3
  CNF3 : Inport  Port=4
  MCP_CNF1 : Constant  Value=hex2dec('2A')  OutDataTypeStr=uint8
  MCP_CNF2 : Constant  Value=hex2dec('29')  OutDataTypeStr=uint8
  MCP_CNF3 : Constant  Value=hex2dec('28')  OutDataTypeStr=uint8
  mcp2515_writeRegister : $bdroot/CAN application/mcp2515 driver CE1/mcp2515_writeRegister  SystemSampleTime=-1
  mcp2515_writeRegister1 : $bdroot/CAN application/mcp2515 driver CE1/mcp2515_writeRegister  SystemSampleTime=-1
  mcp2515_writeRegister2 : $bdroot/CAN application/mcp2515 driver CE1/mcp2515_writeRegister  SystemSampleTime=-1
  Out : Outport
  wires:
  mcp2515_writeRegister2/1 -> Out/1
  mcp2515_writeRegister1/1 -> mcp2515_writeRegister2/1
  mcp2515_writeRegister/1 -> mcp2515_writeRegister1/1
  In/1 -> mcp2515_writeRegister/1
  CNF2/1 -> mcp2515_writeRegister1/3
  MCP_CNF1/1 -> mcp2515_writeRegister/2
  CNF1/1 -> mcp2515_writeRegister/3
  CNF3/1 -> mcp2515_writeRegister2/3
  MCP_CNF3/1 -> mcp2515_writeRegister2/2
  MCP_CNF2/1 -> mcp2515_writeRegister1/2

== system mcp2515lib/CAN application/CANreceive/readRxBuffer/checkRx1Buffer ==
  RX_STATUS : Inport
  Bitmask_RxB1_Status : simulink/Logic and Bit Operations/Bitwise Operator  logicop=AND  UseBitMask=on  BitMask=bin2dec('10000000')  BitMaskRealWorld=Stored Integer
  MCP_READ_RxB0 : Constant  Value=hex2dec('90')  OutDataTypeStr=uint8
  MCP_READ_RxB1 : Constant  Value=hex2dec('94')  OutDataTypeStr=uint8
  Switch : Switch  Criteria=u2 > Threshold
  cmd_read_rx_buff : Outport
  wires:
  RX_STATUS/1 -> Bitmask_RxB1_Status/1
  Bitmask_RxB1_Status/1 -> Switch/2
  MCP_READ_RxB0/1 -> Switch/3
  MCP_READ_RxB1/1 -> Switch/1
  Switch/1 -> cmd_read_rx_buff/1

== system mcp2515lib/CAN application/CANreceive/readRxBuffer/getDLC ==
  RxBx : Inport
  Bitwise Operator : simulink/Logic and Bit Operations/Bitwise Operator  logicop=AND  UseBitMask=off  NumInputPorts=2  BitMask=bin2dec('11011001')  BitMaskRealWorld=Stored Integer
  MCP_DLC_MASK : Constant  Value=hex2dec('0F')  OutDataTypeStr=uint8
  RxDLC : Selector  IndexMode=Zero-based  InputPortWidth=13  IndexOptions=Index vector (dialog)  Indices=4  OutputSizes=1
  CAN_dlc : Outport
  wires:
  MCP_DLC_MASK/1 -> Bitwise Operator/2
  RxDLC/1 -> Bitwise Operator/1
  RxBx/1 -> RxDLC/1
  Bitwise Operator/1 -> CAN_dlc/1

== system mcp2515lib/CAN application/CANreceive/readRxBuffer/getData ==
  RxBx : Inport
  RxData : Selector  IndexMode=Zero-based  InputPortWidth=13  IndexOptions=Index vector (dialog)  Indices=[5:12]  OutputSizes=1
  CAN_data : Outport
  wires:
  RxData/1 -> CAN_data/1
  RxBx/1 -> RxData/1

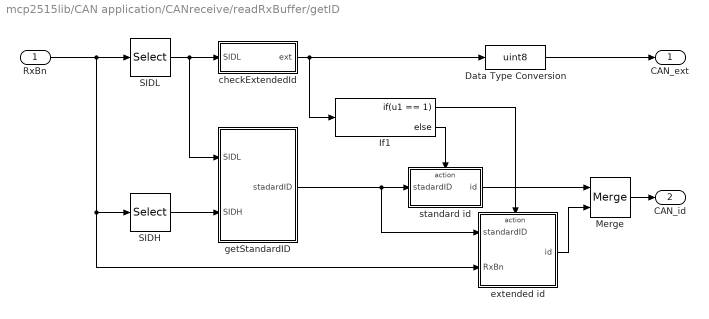
== system mcp2515lib/CAN application/CANreceive/readRxBuffer/getID ==
  RxBn : Inport
  Data Type Conversion : DataTypeConversion  OutDataTypeStr=uint8  RndMeth=Simplest
  If1 : If  IfExpression=u1 == 1
  Merge : Merge
  SIDH : Selector  IndexMode=Zero-based  InputPortWidth=13  IndexOptions=Index vector (dialog)  Indices=0  OutputSizes=1
  SIDL : Selector  IndexMode=Zero-based  InputPortWidth=13  IndexOptions=Index vector (dialog)  Indices=1  OutputSizes=1
  checkExtendedId : Subsystem
  extended id : Subsystem  TreatAsAtomicUnit=on
      settings: RTWSystemCode=Inline
  getStandardID : Subsystem
  standard id : Subsystem  TreatAsAtomicUnit=on
      settings: RTWSystemCode=Inline
  CAN_ext : Outport
  CAN_id : Outport  Port=2
  wires:
  Data Type Conversion/1 -> CAN_ext/1
  checkExtendedId/1(ext) -> If1/1, Data Type Conversion/1
  SIDH/1 -> getStandardID/2(SIDH)
  SIDL/1 -> checkExtendedId/1(SIDL), getStandardID/1(SIDL)
  getStandardID/1(stadardID) -> extended id/1(standardID), standard id/1(stadardID)
  RxBn/1 -> SIDL/1, SIDH/1, extended id/2(RxBn)
  If1/1 -> extended id/Action
  If1/2 -> standard id/Action
  Merge/1 -> CAN_id/1
  extended id/1(id) -> Merge/2
  standard id/1(id) -> Merge/1

== system mcp2515lib/CAN application/CANreceive/readRxBuffer/mcp2515_readRxBuffer ==
  In : Inport
  cmd_read_rx_buff : Inport  Port=2
  Constant : Constant  Value=zeros(1,13)  OutDataTypeStr=uint8
  SPI driver : $bdroot/CAN application/mcp2515 driver/SPI driver  SystemSampleTime=-1
  Selector1 : Selector  IndexMode=Zero-based  InputPortWidth=14  IndexOptions=Index vector (dialog)  Indices=[1:13]  OutputSizes=1
  Vector Concatenate : Concatenate
  Out : Outport
  RxBn : Outport  Port=2
  wires:
  In/1 -> Out/1
  Selector1/1 -> RxBn/1
  SPI driver/1 -> Selector1/1
  Vector Concatenate/1 -> SPI driver/1
  Constant/1 -> Vector Concatenate/2
  cmd_read_rx_buff/1 -> Vector Concatenate/1

== system mcp2515lib/CAN application/CANreceive CE1/readRxBuffer/checkRx1Buffer ==
  RX_STATUS : Inport
  Bitmask_RxB1_Status : simulink/Logic and Bit Operations/Bitwise Operator  logicop=AND  UseBitMask=on  BitMask=bin2dec('10000000')  BitMaskRealWorld=Stored Integer
  MCP_READ_RxB0 : Constant  Value=hex2dec('90')  OutDataTypeStr=uint8
  MCP_READ_RxB1 : Constant  Value=hex2dec('94')  OutDataTypeStr=uint8
  Switch : Switch  Criteria=u2 > Threshold
  cmd_read_rx_buff : Outport
  wires:
  RX_STATUS/1 -> Bitmask_RxB1_Status/1
  Bitmask_RxB1_Status/1 -> Switch/2
  MCP_READ_RxB0/1 -> Switch/3
  MCP_READ_RxB1/1 -> Switch/1
  Switch/1 -> cmd_read_rx_buff/1
